simulink model "LAB5_SIMULINK"  (Simulink 7.3)
settings: Solver=ode45  StartTime=0.0  StopTime=100  RelTol=1e-3
undefined symbols (not defined in the file or in its folder): get
libraries: dspsnks4 x3, dspxfrm3 x2
settings Model: Creator=user_ftk10  LastModifiedBy=user_ftk10

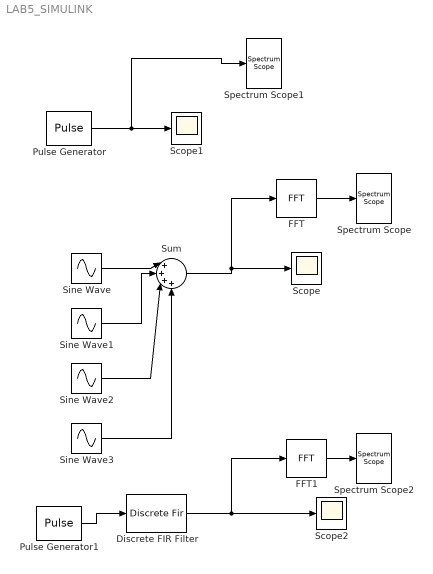
== system LAB5_SIMULINK ==
  Discrete FIR Filter : DiscreteFir  NumCoeffs=ones(1,50)  SampleTime=0.01
  FFT : dspxfrm3/FFT  DialogController=dspDDGCreate  DialogControllerArgs=DataTag0  CompMethod=Table lookup  TableOpt=NEW  TableOptActive=Speed  BitRevOrder=off  InheritFFTLength=on  FFTLength=64  SkipNorm=off  roundingMode=Floor  overflowMode=off
  FFT1 : dspxfrm3/FFT  DialogController=dspDDGCreate  DialogControllerArgs=DataTag1  CompMethod=Table lookup  TableOpt=NEW  TableOptActive=Speed  BitRevOrder=off  InheritFFTLength=on  FFTLength=64  SkipNorm=off  roundingMode=Floor  overflowMode=off
  Pulse Generator : DiscretePulseGenerator  Amplitude=1  Period=100  PulseWidth=50  PhaseDelay=0  SampleTime=0.01
  Pulse Generator1 : DiscretePulseGenerator  Amplitude=1  Period=100  PulseWidth=50  PhaseDelay=0  SampleTime=0.01
  Scope : Scope
  Scope1 : Scope
  Scope2 : Scope
      settings: SaveName=ScopeData2
  Sine Wave : Sin  Amplitude=1  Bias=0  Frequency=2*pi  Phase=0  Samples=10  SampleTime=0.01  Offset=0
  Sine Wave1 : Sin  Amplitude=1  Bias=0  Frequency=4*pi  Phase=0  Samples=10  SampleTime=0.01  Offset=0
  Sine Wave2 : Sin  Amplitude=1  Bias=0  Frequency=6*pi  Phase=0  Samples=10  SampleTime=0.01  Offset=0
  Sine Wave3 : Sin  Amplitude=1  Bias=0  Frequency=8*pi  Phase=0  Samples=10  SampleTime=0.01  Offset=0
  Spectrum Scope : dspsnks4/Spectrum Scope  DialogController=dspdialog.SpectrumScope  DialogControllerArgs=DataTag2  SystemSampleTime=-1  ScopeProperties=on  Domain=Frequency  HorizSpan=1  UseBuffer=on  BufferSize=256  Overlap=128  inpFftLenInherit=off  FFTlength=128  numAvg=2  DisplayProperties=off  AxisGrid=on  Memory=off  FrameNumber=on  AxisLegend=off  AxisZoom=off  OpenScopeAtSimStart=on  OpenScopeImmediately=off  FigPos=get(0,'defaultfigureposition')  AxisProperties=off  XUnits=Hertz  XRange=[0...Fs/2]  XDisplay=0  InheritXIncr=on  XIncr=1.0  XLabel=Samples  XLimit=Auto  YUnits=dB  XMax=1  XMin=0  YLabel=Magnitude-squared, dB  LineProperties=off  wintypeSpecScope=Hann  RsSpecScope=50  betaSpecScope=5  winsampSpecScope=Periodic  XAxisParamsVer=6.9
      settings: YMin=-20  YMax=20
  Spectrum Scope1 : dspsnks4/Spectrum Scope  DialogController=dspdialog.SpectrumScope  DialogControllerArgs=DataTag3  SystemSampleTime=-1  ScopeProperties=on  Domain=Frequency  HorizSpan=1  UseBuffer=on  BufferSize=1024  Overlap=512  inpFftLenInherit=on  FFTlength=512  numAvg=2  DisplayProperties=off  AxisGrid=on  Memory=off  FrameNumber=on  AxisLegend=off  AxisZoom=off  OpenScopeAtSimStart=on  OpenScopeImmediately=off  FigPos=get(0,'defaultfigureposition')  AxisProperties=off  XUnits=Hertz  XRange=[0...Fs/2]  XDisplay=0  InheritXIncr=on  XIncr=1.0  XLabel=Samples  XLimit=Auto  YUnits=dB  XMax=1  XMin=0  YLabel=Magnitude-squared, dB  LineProperties=off  wintypeSpecScope=Hann  RsSpecScope=50  betaSpecScope=5  winsampSpecScope=Periodic  XAxisParamsVer=6.9
      settings: YMin=-200  YMax=200
  Spectrum Scope2 : dspsnks4/Spectrum Scope  DialogController=dspdialog.SpectrumScope  DialogControllerArgs=DataTag4  SystemSampleTime=-1  ScopeProperties=on  Domain=Frequency  HorizSpan=1  UseBuffer=on  BufferSize=256  Overlap=128  inpFftLenInherit=off  FFTlength=128  numAvg=2  DisplayProperties=off  AxisGrid=on  Memory=off  FrameNumber=on  AxisLegend=off  AxisZoom=off  OpenScopeAtSimStart=on  OpenScopeImmediately=off  FigPos=get(0,'defaultfigureposition')  AxisProperties=off  XUnits=Hertz  XRange=[0...Fs/2]  XDisplay=0  InheritXIncr=on  XIncr=1.0  XLabel=Samples  XLimit=Auto  YUnits=dB  XMax=1  XMin=0  YLabel=Magnitude-squared, dB  LineProperties=off  wintypeSpecScope=Hann  RsSpecScope=50  betaSpecScope=5  winsampSpecScope=Periodic  XAxisParamsVer=6.9
      settings: YMin=-20  YMax=20
  Sum : Sum  Inputs=|++++  OutDataType=fixdt(1, 16)  OutScaling=2^0  SampleTime=0.01
  wires:
  Sine Wave/1 -> Sum/1
  Sine Wave1/1 -> Sum/2
  Sum/1 -> Scope/1, FFT/1
  Sine Wave2/1 -> Sum/3
  Sine Wave3/1 -> Sum/4
  FFT/1 -> Spectrum Scope/1
  Pulse Generator/1 -> Scope1/1, Spectrum Scope1/1
  Discrete FIR Filter/1 -> Scope2/1, FFT1/1
  FFT1/1 -> Spectrum Scope2/1
  Pulse Generator1/1 -> Discrete FIR Filter/1
